simulink model "Lowlevel_longitudinal_model"  (R2020a)
settings: Solver=ode45  StartTime=0.0  StopTime=100  FixedStep=0.01  MaxStep=0.001  RelTol=1e-3  EnableMultiTasking=on
InitFcn:
  | %% CACC Simulation Parameters
  | %% by M.Tolga EMIRLER ITU MEKAR
undefined symbols (not defined in the file or in its folder): sigbuilder_block
libraries: simulink x1, simulink_need_slupdate x1
settings Model: Creator=Tolga  LastModifiedBy=apoor
settings DataIOCC: LimitDataPoints=on  SaveFormat=Array  SignalLoggingSaveFormat=ModelDataLogs  ReturnWorkspaceOutputs=off
settings OptimizationCC: ExpressionDepthLimit=2147483647  LifeSpan=inf
settings DebuggingCC: UnderspecifiedInitializationDetection=Classic  MergeDetectMultiDrivingBlocksExec=none  SolverPrmCheckMsg=warning  FcnCallInpInsideContextMsg=warning  StateNameClashWarn=warning  SFUnexpectedBacktrackingDiag=warning  SFNoUnconditionalDefaultTransitionDiag=warning  SFExecutionAtInitializationDiag=none  ArithmeticOperatorsInVariantConditions=warning
settings HardwareCC: ProdBitPerPointer=32  ProdBitPerSizeT=32  ProdBitPerPtrDiffT=32  ProdLargestAtomicFloat=None  ProdIntDivRoundTo=Undefined  ProdEndianess=Unspecified  ProdWordSize=32  ProdHWDeviceType=32-bit Generic
settings ModelReferenceCC: PropagateSignalLabelsOutOfModel=off
settings SFSimCC: SimUseLocalCustomCode=off  CustomCodeUndefinedFunction=UseInterfaceOnly
settings RTWCC: RTWUseLocalCustomCode=off
settings CodeAppCC: StateflowObjectComments=on
settings GRTTargetCC: TargetLangStandard=C89/C90 (ANSI)  CombineOutputUpdateFcns=off  GRTInterface=on
settings ConfigComp: CovMetricSettings=dw  CovHtmlReporting=on  CovSaveCumulativeToWorkspaceVar=on  CovSaveSingleToWorkspaceVar=on  CovExternalEMLEnable=off  CovSFcnEnable=off

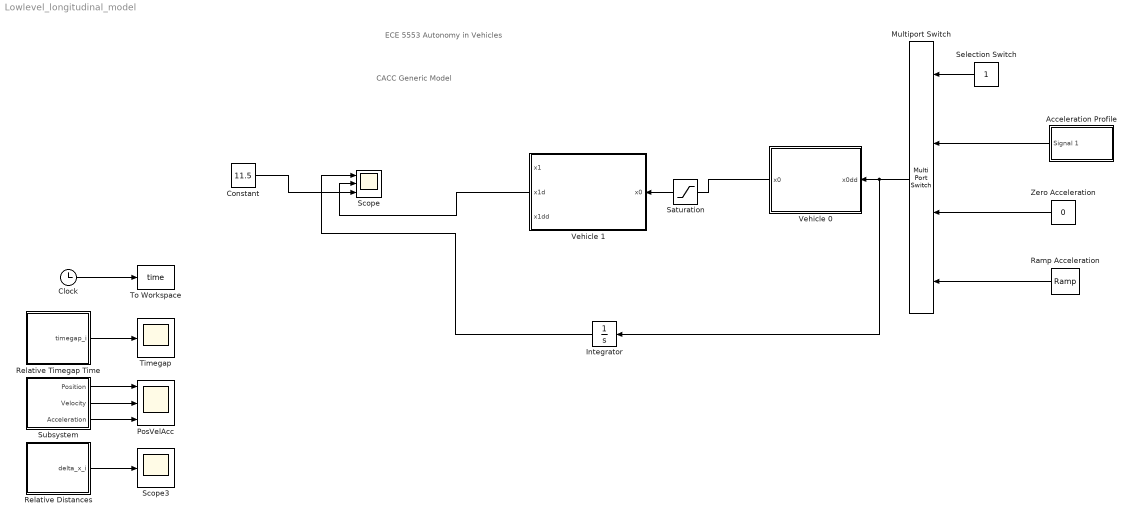
== system Lowlevel_longitudinal_model ==
  note: ECE 5553 Autonomy in Vehicles
  note: CACC Generic Model
  Acceleration Profile : Subsystem  Tag=STV Subsys  LoadFcn=sigbuilder_block('load');  StartFcn=sigbuilder_block('start');  StopFcn=sigbuilder_block('stop');  ClipboardFcn=sigbuilder_block('clipboard');  mask(Sigbuilder block){tuvar=[0:10]}
      mask help: Sigbuilder GUI
      mask init:
      | if ~strcmp(get_param(bdroot(gcbh),'SimulationStatus'),'stopped') tuvar = sigbuilder_block('maskInit'); end
      settings: CopyFcn=sigbuilder_block('copy');  DeleteFcn=sigbuilder_block('delete');  ModelCloseFcn=sigbuilder_block('modelClose');  PreSaveFcn=sigbuilder_block('preSave');  PauseFcn=sigbuilder_block('pause')  ContinueFcn=sigbuilder_block('continue')  NameChangeFcn=sigbuilder_block('namechange');  OpenFcn=sigbuilder_block('open',[386.25 100.5 510.75 487.5 ]);  CloseFcn=sigbuilder_block('close');
      mask Display: plot(0, 0, 100, 100,[2, 2, 32, 32, 2], [68, 8, 8, 68, 68],[32, 2], [38, 38], [32, 19, 2],[53, 60, 44], [32, 17, 17, 2],[16, 16, 31, 31]);txt = getActiveGroup(gcbh);text(2, 100, txt,'verticalAlignment', 'top');
  Clock : Clock
  Constant : Constant  Value=11.5
  Integrator : Integrator
  Multiport Switch : MultiPortSwitch
  PosVelAcc : Scope  NumInputPorts=3
  Ramp Acceleration : simulink/Sources/Ramp  slope=1  start=0  InitialOutput=40
  Relative Distances : Subsystem
  Relative Timegap Time : Subsystem
  Saturation : Saturate  UpperLimit=11
  Scope : Scope  NumInputPorts=3
  Scope3 : Scope
  Selection Switch : Constant
  Subsystem : Subsystem
  Timegap : Scope
  To Workspace : ToWorkspace  VariableName=time  SampleTime=-1
  Vehicle 0 : Subsystem  mask(INPUT BLOCK){x0in=211, V0in=0}
      mask prompts: x0in "Initial position (x0in)"; V0in "Initial velocity (V0in)"
      mask help: This block defines the input. Input (or disturbance) is the acceleration.
      mask Display:
      | disp('Input')
      | port_label('input',1,'a0')
      | port_label('output',1,'x0')
  Vehicle 1 : Subsystem  mask(VEHICLE #1 (GCDC Vehicle)){kG1=1.0, T1=0.5, phi1=0.1, theta1=0.3, hd1=0.6, L1=5, r1=30, x1in=176, V1in=0, CACC1=1, wK1=2.4}
      mask prompts: kG1 "Vehicle Model Gain (kG1)"; T1 "Vehicle Time Constant (T1)"; phi1 "Actuator (Internal) Delay (phi1) [s]"; theta1 "Communication System Delay (theta1) [s]"; hd1 "Headway time (hd1) [s]"; L1 "Vehicle length (L1) [m]"; r1 "Distance at standstill (r1) [m]"; x1in "Initial vehicle position (x1in) [m]"; V1in "Initial vehicle velocity (V1in) [m/sec]"; CACC1 "CACC On/Off [0 or 1]"; wK1 "Controller Gain (wK1)"
      mask help: Parameters for vehicle 1
      mask Display:
      | disp('Vehicle 1')
      | port_label('input',1,'x0')
      | port_label('output',1,'x1')
      | port_label('output',2,'V1')
      | port_label('output',3,'a1')
  Zero Acceleration : Constant  Value=0
  wires:
  Clock/1 -> To Workspace/1
  Relative Distances/1(delta_x_i) -> Scope3/1
  Vehicle 0/1(x0) -> Vehicle 1/1(x0)
  Ramp Acceleration/1 -> Multiport Switch/4
  Zero Acceleration/1 -> Multiport Switch/3
  Relative Timegap Time/1(timegap_i) -> Timegap/1
  Selection Switch/1 -> Multiport Switch/1
  Multiport Switch/1 -> Integrator/1, Vehicle 0/1(x0dd)
  Subsystem/1(Position) -> PosVelAcc/1
  Subsystem/2(Velocity) -> PosVelAcc/2
  Subsystem/3(Acceleration) -> PosVelAcc/3
  Vehicle 1/2(x1d) -> Scope/2
  Integrator/1 -> Scope/1
  Acceleration Profile/1(Signal 1) -> Multiport Switch/2
  Constant/1 -> Scope/3

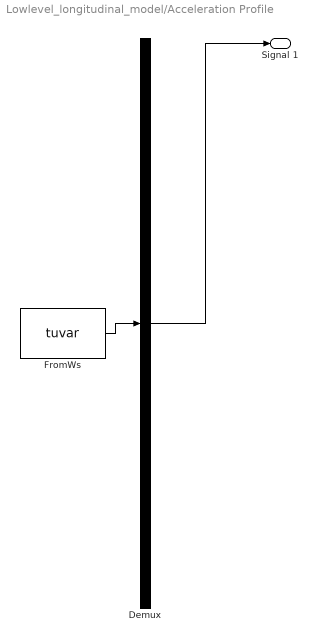
== system Lowlevel_longitudinal_model/Acceleration Profile ==
  Demux : Demux  Tag=STV Demux  Outputs=1
      settings: DisplayOption=none
  FromWs : FromWorkspace  Tag=STV FromWs  VariableName=tuvar
      SigBuilderData=|
      | common.afterFinalStr = 'Extrapolate'
      | common.sampleTime = 0
      | dataSet.timeRange = [0 50]
      | dataSet.name = 'Group 1'
      | sbobj.Groups.Name = 'Group 1'
      | sbobj.Groups.Signals.Name = 'Signal 1'
      | sbobj.Groups.Signals.XData = [0 5 10 15 25 30 35 40 50]
      | sbobj.Groups.Signals.YData = [0 1 1 0 0 -1 -1 0 0]
      | sbobj.Groups.TimeRange = [0 50]
  Signal 1 : Outport  Tag=STV Outport  VectorParamsAs1DForOutWhenUnconnected=off
  wires:
  Demux/1 -> Signal 1/1
  FromWs/1 -> Demux/1

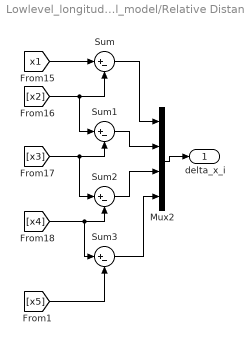
== system Lowlevel_longitudinal_model/Relative Distances ==
  Mux2 : Mux
  Sum{,1..3} (4 alike) : Sum  Inputs=|+-
  delta_x_i : Outport  VectorParamsAs1DForOutWhenUnconnected=off
  wires:
  [x1] -> Sum/1
  [x2] -> Sum/2, Sum1/1
  [x3] -> Sum1/2, Sum2/1
  Sum/1 -> Mux2/1
  Sum1/1 -> Mux2/2
  Sum2/1 -> Mux2/3
  Mux2/1 -> delta_x_i/1
  Sum3/1 -> Mux2/4
  [x5] -> Sum3/2
  [x4] -> Sum3/1, Sum2/2

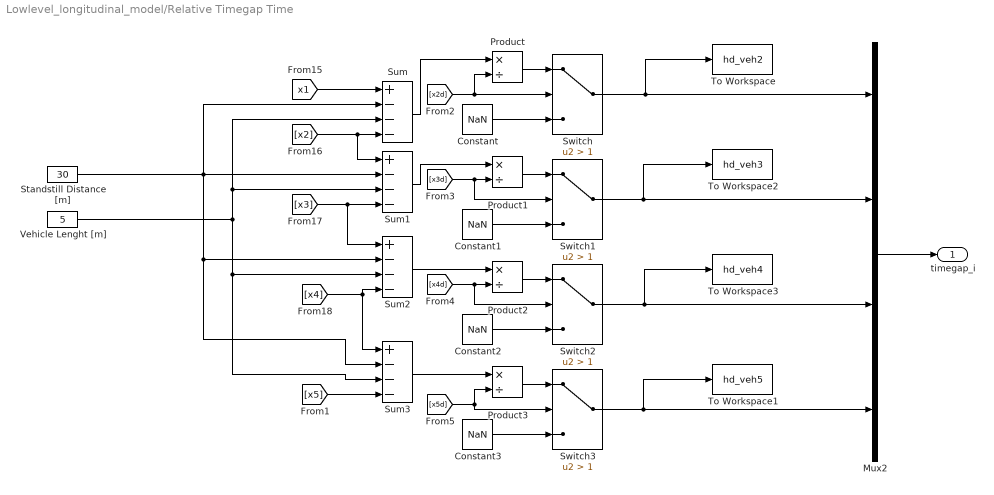
== system Lowlevel_longitudinal_model/Relative Timegap Time ==
  Constant{,1..3} (4 alike) : Constant  Value=NaN
  Mux2 : Mux
  Product{,1..3} (4 alike) : Product  Inputs=*/
  Standstill Distance [m] : Constant  Value=30
  Sum{,1..3} (4 alike) : Sum  Inputs=+---
  Switch{,1..3} (4 alike) : Switch  Criteria=u2 > Threshold  Threshold=1
  To Workspace : ToWorkspace  VariableName=hd_veh2  SampleTime=-1
  To Workspace1 : ToWorkspace  VariableName=hd_veh5  SampleTime=-1
  To Workspace2 : ToWorkspace  VariableName=hd_veh3  SampleTime=-1
  To Workspace3 : ToWorkspace  VariableName=hd_veh4  SampleTime=-1
  Vehicle Lenght [m] : Constant  Value=5
  timegap_i : Outport  VectorParamsAs1DForOutWhenUnconnected=off
  wires:
  [x4] -> Sum3/1, Sum2/4
  [x5] -> Sum3/4
  Mux2/1 -> timegap_i/1
  Sum/1 -> Product/1
  [x3] -> Sum2/1, Sum1/4
  [x2] -> Sum1/1, Sum/4
  [x1] -> Sum/1
  Product/1 -> Switch/1
  [x2d] -> Switch/2, Product/2
  Constant/1 -> Switch/3
  Switch/1 -> Mux2/1, To Workspace/1
  Constant1/1 -> Switch1/3
  [x3d] -> Switch1/2, Product1/2
  Product1/1 -> Switch1/1
  Sum1/1 -> Product1/1
  Sum2/1 -> Product2/1
  Product2/1 -> Switch2/1
  [x4d] -> Switch2/2, Product2/2
  Constant2/1 -> Switch2/3
  Constant3/1 -> Switch3/3
  [x5d] -> Switch3/2, Product3/2
  Product3/1 -> Switch3/1
  Sum3/1 -> Product3/1
  Switch1/1 -> To Workspace2/1, Mux2/2
  Switch3/1 -> To Workspace1/1, Mux2/4
  Switch2/1 -> To Workspace3/1, Mux2/3
  Standstill Distance [m]/1 -> Sum3/2, Sum2/2, Sum1/2, Sum/2
  Vehicle Lenght [m]/1 -> Sum3/3, Sum2/3, Sum1/3, Sum/3

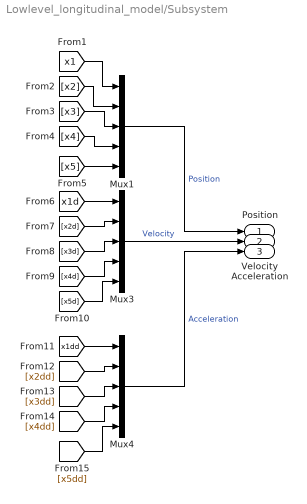
== system Lowlevel_longitudinal_model/Subsystem ==
  Mux1 : Mux  Inputs=5
  Mux3 : Mux  Inputs=5
  Mux4 : Mux  Inputs=5
  Position : Outport  VectorParamsAs1DForOutWhenUnconnected=off
  Velocity : Outport  Port=2  VectorParamsAs1DForOutWhenUnconnected=off
  Acceleration : Outport  Port=3  VectorParamsAs1DForOutWhenUnconnected=off
  wires:
  Mux1/1 -> Position/1  "Position"
  Mux3/1 -> Velocity/1  "Velocity"
  Mux4/1 -> Acceleration/1  "Acceleration"
  [x2dd] -> Mux4/2
  [x2] -> Mux1/2
  [x1dd] -> Mux4/1
  [x4d] -> Mux3/4
  [x1] -> Mux1/1
  [x4] -> Mux1/4
  [x1d] -> Mux3/1
  [x3d] -> Mux3/3
  [x4dd] -> Mux4/4
  [x3] -> Mux1/3
  [x2d] -> Mux3/2
  [x3dd] -> Mux4/3
  [x5dd] -> Mux4/5
  [x5d] -> Mux3/5
  [x5] -> Mux1/5

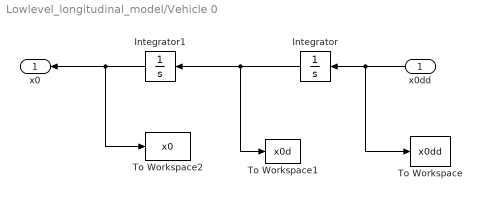
== system Lowlevel_longitudinal_model/Vehicle 0 ==
  x0dd : Inport
  Integrator : Integrator  InitialCondition=V0in
  Integrator1 : Integrator  InitialCondition=x0in
  To Workspace : ToWorkspace  VariableName=x0dd  SampleTime=-1
  To Workspace1 : ToWorkspace  VariableName=x0d  SampleTime=-1
  To Workspace2 : ToWorkspace  VariableName=x0  SampleTime=-1
  x0 : Outport  VectorParamsAs1DForOutWhenUnconnected=off
  wires:
  Integrator/1 -> Integrator1/1, To Workspace1/1
  x0dd/1 -> Integrator/1, To Workspace/1
  Integrator1/1 -> x0/1, To Workspace2/1

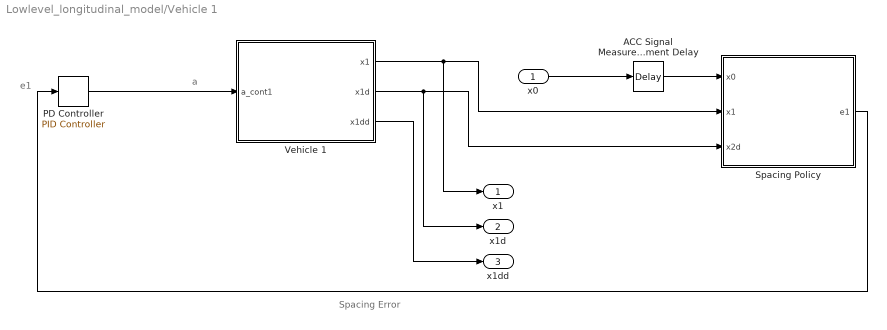
== system Lowlevel_longitudinal_model/Vehicle 1 ==
  note: a
  note: e1
  note: Spacing Error
  x0 : Inport
  ACC Signal Measurement Delay : TransportDelay  DelayTime=0
  PD Controller : simulink_need_slupdate/PID Controller  P=wK1^2  I=0  D=wK1
  Spacing Policy : Subsystem
  Vehicle 1 : Subsystem
  x1 : Outport  VectorParamsAs1DForOutWhenUnconnected=off
  x1d : Outport  Port=2  VectorParamsAs1DForOutWhenUnconnected=off
  x1dd : Outport  Port=3  VectorParamsAs1DForOutWhenUnconnected=off
  wires:
  Vehicle 1/3(x1dd) -> x1dd/1
  Vehicle 1/2(x1d) -> x1d/1, Spacing Policy/3(x2d)
  Vehicle 1/1(x1) -> x1/1, Spacing Policy/2(x1)
  Spacing Policy/1(e1) -> PD Controller/1
  x0/1 -> ACC Signal Measurement Delay/1
  PD Controller/1 -> Vehicle 1/1(a_cont1)
  ACC Signal Measurement Delay/1 -> Spacing Policy/1(x0)

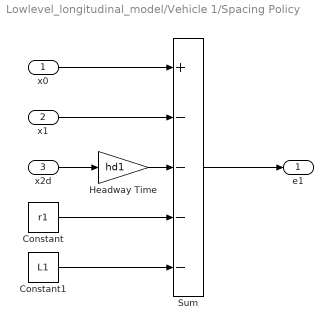
== system Lowlevel_longitudinal_model/Vehicle 1/Spacing Policy ==
  x0 : Inport
  x1 : Inport  Port=2
  x2d : Inport  Port=3
  Constant : Constant  Value=r1
  Constant1 : Constant  Value=L1
  Headway Time : Gain  Gain=hd1
  Sum : Sum  Inputs=+----
  e1 : Outport  VectorParamsAs1DForOutWhenUnconnected=off
  wires:
  x2d/1 -> Headway Time/1
  Headway Time/1 -> Sum/3
  Sum/1 -> e1/1
  x1/1 -> Sum/2
  x0/1 -> Sum/1
  Constant1/1 -> Sum/5
  Constant/1 -> Sum/4

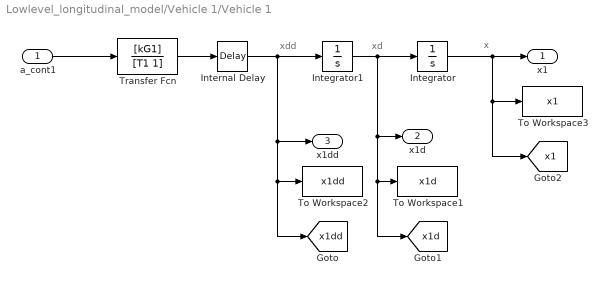
== system Lowlevel_longitudinal_model/Vehicle 1/Vehicle 1 ==
  note: xdd
  note: xd
  note: x
  a_cont1 : Inport
  Integrator : Integrator  InitialCondition=x1in
  Integrator1 : Integrator  InitialCondition=V1in
  Internal Delay : TransportDelay  DelayTime=phi1
  To Workspace1 : ToWorkspace  VariableName=x1d  SampleTime=-1
  To Workspace2 : ToWorkspace  VariableName=x1dd  SampleTime=-1
  To Workspace3 : ToWorkspace  VariableName=x1  SampleTime=-1
  Transfer Fcn : TransferFcn  Numerator=[kG1]  Denominator=[T1 1]
  x1 : Outport  VectorParamsAs1DForOutWhenUnconnected=off
  x1d : Outport  Port=2  VectorParamsAs1DForOutWhenUnconnected=off
  x1dd : Outport  Port=3  VectorParamsAs1DForOutWhenUnconnected=off
  tag scope: x1=global, x1d=global, x1dd=global
  wires:
  Integrator/1 -> [x1], To Workspace3/1, x1/1
  a_cont1/1 -> Transfer Fcn/1
  Transfer Fcn/1 -> Internal Delay/1
  Internal Delay/1 -> [x1dd], To Workspace2/1, x1dd/1, Integrator1/1
  Integrator1/1 -> [x1d], To Workspace1/1, x1d/1, Integrator/1
